simulink model "Dynamics"  (R2023a)
settings: Solver=FixedStepAuto  StartTime=0.0  StopTime=inf  FixedStep=0.001  EnableMultiTasking=on
libraries: sharedutil x32, sharedtransform x18, dspmtrx3 x12, matrix_library x6, simulink_extras x1, simulink x1
(part 4 of 6)

== system Dynamics/Subsystem2/Jacobian/J(q) gen./J_v_2(q) ==
  R_1^0 : Inport
  p_1^0 : Inport  Port=2
  p_2^0 : Inport  Port=3
  type1 : Inport  Port=4
  Constant : Constant  Value=zeros(3,1)
  J_v_1 : Subsystem
  v2M_1 : MATLAB Function  TreatAsAtomicUnit=on
  v2M_2 : MATLAB Function  TreatAsAtomicUnit=on
  v2M_3 : MATLAB Function  TreatAsAtomicUnit=on
  v2M_4 : MATLAB Function  TreatAsAtomicUnit=on
  v2M_5 : MATLAB Function  TreatAsAtomicUnit=on
  J_v_2(q) : Outport
  wires:
  R_1^0/1 -> J_v_1/1(R)
  J_v_1/1(J_v) -> v2M_1/1(v1)
  v2M_1/1(M) -> v2M_2/1(v1)
  v2M_2/1(M) -> v2M_3/1(v1)
  v2M_3/1(M) -> v2M_4/1(v1)
  v2M_4/1(M) -> v2M_5/1(v1)
  v2M_5/1(M) -> J_v_2(q)/1
  Constant/1 -> v2M_3/2(v2), v2M_4/2(v2), v2M_5/2(v2), v2M_1/2(v2), v2M_2/2(v2)
  p_1^0/1 -> J_v_1/2(p)
  type1/1 -> J_v_1/4(type)
  p_2^0/1 -> J_v_1/3(pn)

== system Dynamics/Subsystem2/Jacobian/J(q) gen./J_v_3(q) ==
  R_1^0 : Inport
  R_2^0 : Inport  Port=2
  p_1^0 : Inport  Port=3
  p_2^0 : Inport  Port=4
  p_3^0 : Inport  Port=5
  type1 : Inport  Port=6
  type2 : Inport  Port=7
  Constant : Constant  Value=zeros(3,1)
  J_v_1 : Subsystem
  J_v_2 : Subsystem
  v2M_1 : MATLAB Function  TreatAsAtomicUnit=on
  v2M_2 : MATLAB Function  TreatAsAtomicUnit=on
  v2M_3 : MATLAB Function  TreatAsAtomicUnit=on
  v2M_4 : MATLAB Function  TreatAsAtomicUnit=on
  v2M_5 : MATLAB Function  TreatAsAtomicUnit=on
  J_v_3(q) : Outport
  wires:
  R_1^0/1 -> J_v_1/1(R)
  J_v_1/1(J_v) -> v2M_1/1(v1)
  v2M_1/1(M) -> v2M_2/1(v1)
  v2M_2/1(M) -> v2M_3/1(v1)
  v2M_3/1(M) -> v2M_4/1(v1)
  v2M_4/1(M) -> v2M_5/1(v1)
  v2M_5/1(M) -> J_v_3(q)/1
  J_v_2/1(J_v) -> v2M_1/2(v2)
  Constant/1 -> v2M_5/2(v2), v2M_4/2(v2), v2M_2/2(v2), v2M_3/2(v2)
  R_2^0/1 -> J_v_2/1(R)
  p_1^0/1 -> J_v_1/2(p)
  p_2^0/1 -> J_v_2/2(p)
  type2/1 -> J_v_2/4(type)
  type1/1 -> J_v_1/4(type)
  p_3^0/1 -> J_v_1/3(pn), J_v_2/3(pn)

== system Dynamics/Subsystem2/Jacobian/J(q) gen./J_v_4(q) ==
  R_1^0 : Inport
  R_2^0 : Inport  Port=2
  R_3^0 : Inport  Port=3
  p_1^0 : Inport  Port=4
  p_2^0 : Inport  Port=5
  p_3^0 : Inport  Port=6
  p_4^0 : Inport  Port=7
  type1 : Inport  Port=8
  type2 : Inport  Port=9
  type3 : Inport  Port=10
  Constant : Constant  Value=zeros(3,1)
  J_v_1 : Subsystem
  J_v_2 : Subsystem
  J_v_3 : Subsystem
  v2M_1 : MATLAB Function  TreatAsAtomicUnit=on
  v2M_2 : MATLAB Function  TreatAsAtomicUnit=on
  v2M_3 : MATLAB Function  TreatAsAtomicUnit=on
  v2M_4 : MATLAB Function  TreatAsAtomicUnit=on
  v2M_5 : MATLAB Function  TreatAsAtomicUnit=on
  J_v_4(q) : Outport
  wires:
  R_1^0/1 -> J_v_1/1(R)
  J_v_1/1(J_v) -> v2M_1/1(v1)
  v2M_1/1(M) -> v2M_2/1(v1)
  v2M_2/1(M) -> v2M_3/1(v1)
  v2M_3/1(M) -> v2M_4/1(v1)
  v2M_4/1(M) -> v2M_5/1(v1)
  v2M_5/1(M) -> J_v_4(q)/1
  J_v_2/1(J_v) -> v2M_1/2(v2)
  J_v_3/1(J_v) -> v2M_2/2(v2)
  Constant/1 -> v2M_5/2(v2), v2M_3/2(v2), v2M_4/2(v2)
  R_2^0/1 -> J_v_2/1(R)
  R_3^0/1 -> J_v_3/1(R)
  p_1^0/1 -> J_v_1/2(p)
  p_2^0/1 -> J_v_2/2(p)
  p_3^0/1 -> J_v_3/2(p)
  type2/1 -> J_v_2/4(type)
  type1/1 -> J_v_1/4(type)
  type3/1 -> J_v_3/4(type)
  p_4^0/1 -> J_v_1/3(pn), J_v_2/3(pn), J_v_3/3(pn)

== system Dynamics/Subsystem2/Jacobian/J(q) gen./J_v_5(q) ==
  R_1^0 : Inport
  R_2^0 : Inport  Port=2
  R_3^0 : Inport  Port=3
  R_4^0 : Inport  Port=4
  p_1^0 : Inport  Port=5
  p_2^0 : Inport  Port=6
  p_3^0 : Inport  Port=7
  p_4^0 : Inport  Port=8
  p_5^0 : Inport  Port=9
  type1 : Inport  Port=10
  type2 : Inport  Port=11
  type3 : Inport  Port=12
  type4 : Inport  Port=13
  Constant : Constant  Value=zeros(3,1)
  J_v_1 : Subsystem
  J_v_2 : Subsystem
  J_v_3 : Subsystem
  J_v_4 : Subsystem
  v2M_1 : MATLAB Function  TreatAsAtomicUnit=on
  v2M_2 : MATLAB Function  TreatAsAtomicUnit=on
  v2M_3 : MATLAB Function  TreatAsAtomicUnit=on
  v2M_4 : MATLAB Function  TreatAsAtomicUnit=on
  v2M_5 : MATLAB Function  TreatAsAtomicUnit=on
  J_v_5(q) : Outport
  wires:
  R_1^0/1 -> J_v_1/1(R)
  J_v_1/1(J_v) -> v2M_1/1(v1)
  v2M_1/1(M) -> v2M_2/1(v1)
  v2M_2/1(M) -> v2M_3/1(v1)
  v2M_3/1(M) -> v2M_4/1(v1)
  v2M_4/1(M) -> v2M_5/1(v1)
  v2M_5/1(M) -> J_v_5(q)/1
  J_v_2/1(J_v) -> v2M_1/2(v2)
  J_v_3/1(J_v) -> v2M_2/2(v2)
  J_v_4/1(J_v) -> v2M_3/2(v2)
  Constant/1 -> v2M_4/2(v2), v2M_5/2(v2)
  R_2^0/1 -> J_v_2/1(R)
  R_3^0/1 -> J_v_3/1(R)
  R_4^0/1 -> J_v_4/1(R)
  p_1^0/1 -> J_v_1/2(p)
  p_2^0/1 -> J_v_2/2(p)
  p_3^0/1 -> J_v_3/2(p)
  p_4^0/1 -> J_v_4/2(p)
  type2/1 -> J_v_2/4(type)
  type1/1 -> J_v_1/4(type)
  type3/1 -> J_v_3/4(type)
  type4/1 -> J_v_4/4(type)
  p_5^0/1 -> J_v_1/3(pn), J_v_2/3(pn), J_v_3/3(pn), J_v_4/3(pn)

== system Dynamics/Subsystem2/Jacobian/J_v/J_v_1 ==
  R : Inport
  p : Inport  Port=2
  pn : Inport  Port=3
  type : Inport  Port=4
  Add : Sum
  If : If  IfExpression=u1 == 1
  Prismatic Action : Subsystem  TreatAsAtomicUnit=on
  Revolute Action : Subsystem  TreatAsAtomicUnit=on
  J_v : Outport
  wires:
  type/1 -> If/1
  If/1 -> Revolute Action/Action
  If/2 -> Prismatic Action/Action
  Revolute Action/1(J_v) -> Add/1
  Prismatic Action/1(J_v) -> Add/2
  Add/1 -> J_v/1
  R/1 -> Prismatic Action/1(R), Revolute Action/1(R)
  p/1 -> Revolute Action/2(p)
  pn/1 -> Revolute Action/3(pn)

== system Dynamics/Subsystem2/Jacobian/J_v/J_v_2 ==
  R : Inport
  p : Inport  Port=2
  pn : Inport  Port=3
  type : Inport  Port=4
  Add : Sum
  If : If  IfExpression=u1 == 1
  Prismatic Action : Subsystem  TreatAsAtomicUnit=on
  Revolute Action : Subsystem  TreatAsAtomicUnit=on
  J_v : Outport
  wires:
  type/1 -> If/1
  If/1 -> Revolute Action/Action
  If/2 -> Prismatic Action/Action
  Revolute Action/1(J_v) -> Add/1
  Prismatic Action/1(J_v) -> Add/2
  Add/1 -> J_v/1
  R/1 -> Prismatic Action/1(R), Revolute Action/1(R)
  p/1 -> Revolute Action/2(p)
  pn/1 -> Revolute Action/3(pn)

== system Dynamics/Subsystem2/Jacobian/J_v/J_v_3 ==
  R : Inport
  p : Inport  Port=2
  pn : Inport  Port=3
  type : Inport  Port=4
  Add : Sum
  If : If  IfExpression=u1 == 1
  Prismatic Action : Subsystem  TreatAsAtomicUnit=on
  Revolute Action : Subsystem  TreatAsAtomicUnit=on
  J_v : Outport
  wires:
  type/1 -> If/1
  If/1 -> Revolute Action/Action
  If/2 -> Prismatic Action/Action
  Revolute Action/1(J_v) -> Add/1
  Prismatic Action/1(J_v) -> Add/2
  Add/1 -> J_v/1
  R/1 -> Prismatic Action/1(R), Revolute Action/1(R)
  p/1 -> Revolute Action/2(p)
  pn/1 -> Revolute Action/3(pn)

== system Dynamics/Subsystem2/Jacobian/J_v/J_v_4 ==
  R : Inport
  p : Inport  Port=2
  pn : Inport  Port=3
  type : Inport  Port=4
  Add : Sum
  If : If  IfExpression=u1 == 1
  Prismatic Action : Subsystem  TreatAsAtomicUnit=on
  Revolute Action : Subsystem  TreatAsAtomicUnit=on
  J_v : Outport
  wires:
  type/1 -> If/1
  If/1 -> Revolute Action/Action
  If/2 -> Prismatic Action/Action
  Revolute Action/1(J_v) -> Add/1
  Prismatic Action/1(J_v) -> Add/2
  Add/1 -> J_v/1
  R/1 -> Prismatic Action/1(R), Revolute Action/1(R)
  p/1 -> Revolute Action/2(p)
  pn/1 -> Revolute Action/3(pn)

== system Dynamics/Subsystem2/Jacobian/J_v/J_v_5 ==
  R : Inport
  p : Inport  Port=2
  pn : Inport  Port=3
  type : Inport  Port=4
  Add : Sum
  If : If  IfExpression=u1 == 1
  Prismatic Action : Subsystem  TreatAsAtomicUnit=on
  Revolute Action : Subsystem  TreatAsAtomicUnit=on
  J_v : Outport
  wires:
  type/1 -> If/1
  If/1 -> Revolute Action/Action
  If/2 -> Prismatic Action/Action
  Revolute Action/1(J_v) -> Add/1
  Prismatic Action/1(J_v) -> Add/2
  Add/1 -> J_v/1
  R/1 -> Prismatic Action/1(R), Revolute Action/1(R)
  p/1 -> Revolute Action/2(p)
  pn/1 -> Revolute Action/3(pn)

== system Dynamics/Subsystem2/Jacobian/J_v/J_v_6 ==
  R : Inport
  p : Inport  Port=2
  pn : Inport  Port=3
  type : Inport  Port=4
  Add : Sum
  If : If  IfExpression=u1 == 1
  Prismatic Action : Subsystem  TreatAsAtomicUnit=on
  Revolute Action : Subsystem  TreatAsAtomicUnit=on
  J_v : Outport
  wires:
  type/1 -> If/1
  If/1 -> Revolute Action/Action
  If/2 -> Prismatic Action/Action
  Revolute Action/1(J_v) -> Add/1
  Prismatic Action/1(J_v) -> Add/2
  Add/1 -> J_v/1
  R/1 -> Prismatic Action/1(R), Revolute Action/1(R)
  p/1 -> Revolute Action/2(p)
  pn/1 -> Revolute Action/3(pn)

== system Dynamics/DYNAMIC/Jacobian/J(q) gen./J_v_2(q)/J_v_1 ==
  R : Inport
  p : Inport  Port=2
  pn : Inport  Port=3
  type : Inport  Port=4
  Add : Sum
  If : If  IfExpression=u1 == 1
  Prismatic Action : Subsystem  TreatAsAtomicUnit=on
  Revolute Action : Subsystem  TreatAsAtomicUnit=on
  J_v : Outport
  wires:
  type/1 -> If/1
  If/1 -> Revolute Action/Action
  If/2 -> Prismatic Action/Action
  Revolute Action/1(J_v) -> Add/1
  Prismatic Action/1(J_v) -> Add/2
  Add/1 -> J_v/1
  R/1 -> Prismatic Action/1(R), Revolute Action/1(R)
  p/1 -> Revolute Action/2(p)
  pn/1 -> Revolute Action/3(pn)

== system Dynamics/DYNAMIC/Jacobian/J(q) gen./J_v_3(q)/J_v_1 ==
  R : Inport
  p : Inport  Port=2
  pn : Inport  Port=3
  type : Inport  Port=4
  Add : Sum
  If : If  IfExpression=u1 == 1
  Prismatic Action : Subsystem  TreatAsAtomicUnit=on
  Revolute Action : Subsystem  TreatAsAtomicUnit=on
  J_v : Outport
  wires:
  type/1 -> If/1
  If/1 -> Revolute Action/Action
  If/2 -> Prismatic Action/Action
  Revolute Action/1(J_v) -> Add/1
  Prismatic Action/1(J_v) -> Add/2
  Add/1 -> J_v/1
  R/1 -> Prismatic Action/1(R), Revolute Action/1(R)
  p/1 -> Revolute Action/2(p)
  pn/1 -> Revolute Action/3(pn)

== system Dynamics/DYNAMIC/Jacobian/J(q) gen./J_v_3(q)/J_v_2 ==
  R : Inport
  p : Inport  Port=2
  pn : Inport  Port=3
  type : Inport  Port=4
  Add : Sum
  If : If  IfExpression=u1 == 1
  Prismatic Action : Subsystem  TreatAsAtomicUnit=on
  Revolute Action : Subsystem  TreatAsAtomicUnit=on
  J_v : Outport
  wires:
  type/1 -> If/1
  If/1 -> Revolute Action/Action
  If/2 -> Prismatic Action/Action
  Revolute Action/1(J_v) -> Add/1
  Prismatic Action/1(J_v) -> Add/2
  Add/1 -> J_v/1
  R/1 -> Prismatic Action/1(R), Revolute Action/1(R)
  p/1 -> Revolute Action/2(p)
  pn/1 -> Revolute Action/3(pn)

== system Dynamics/DYNAMIC/Jacobian/J(q) gen./J_v_4(q)/J_v_1 ==
  R : Inport
  p : Inport  Port=2
  pn : Inport  Port=3
  type : Inport  Port=4
  Add : Sum
  If : If  IfExpression=u1 == 1
  Prismatic Action : Subsystem  TreatAsAtomicUnit=on
  Revolute Action : Subsystem  TreatAsAtomicUnit=on
  J_v : Outport
  wires:
  type/1 -> If/1
  If/1 -> Revolute Action/Action
  If/2 -> Prismatic Action/Action
  Revolute Action/1(J_v) -> Add/1
  Prismatic Action/1(J_v) -> Add/2
  Add/1 -> J_v/1
  R/1 -> Prismatic Action/1(R), Revolute Action/1(R)
  p/1 -> Revolute Action/2(p)
  pn/1 -> Revolute Action/3(pn)

== system Dynamics/DYNAMIC/Jacobian/J(q) gen./J_v_4(q)/J_v_2 ==
  R : Inport
  p : Inport  Port=2
  pn : Inport  Port=3
  type : Inport  Port=4
  Add : Sum
  If : If  IfExpression=u1 == 1
  Prismatic Action : Subsystem  TreatAsAtomicUnit=on
  Revolute Action : Subsystem  TreatAsAtomicUnit=on
  J_v : Outport
  wires:
  type/1 -> If/1
  If/1 -> Revolute Action/Action
  If/2 -> Prismatic Action/Action
  Revolute Action/1(J_v) -> Add/1
  Prismatic Action/1(J_v) -> Add/2
  Add/1 -> J_v/1
  R/1 -> Prismatic Action/1(R), Revolute Action/1(R)
  p/1 -> Revolute Action/2(p)
  pn/1 -> Revolute Action/3(pn)

== system Dynamics/DYNAMIC/Jacobian/J(q) gen./J_v_4(q)/J_v_3 ==
  R : Inport
  p : Inport  Port=2
  pn : Inport  Port=3
  type : Inport  Port=4
  Add : Sum
  If : If  IfExpression=u1 == 1
  Prismatic Action : Subsystem  TreatAsAtomicUnit=on
  Revolute Action : Subsystem  TreatAsAtomicUnit=on
  J_v : Outport
  wires:
  type/1 -> If/1
  If/1 -> Revolute Action/Action
  If/2 -> Prismatic Action/Action
  Revolute Action/1(J_v) -> Add/1
  Prismatic Action/1(J_v) -> Add/2
  Add/1 -> J_v/1
  R/1 -> Prismatic Action/1(R), Revolute Action/1(R)
  p/1 -> Revolute Action/2(p)
  pn/1 -> Revolute Action/3(pn)

== system Dynamics/DYNAMIC/Jacobian/J(q) gen./J_v_5(q)/J_v_1 ==
  R : Inport
  p : Inport  Port=2
  pn : Inport  Port=3
  type : Inport  Port=4
  Add : Sum
  If : If  IfExpression=u1 == 1
  Prismatic Action : Subsystem  TreatAsAtomicUnit=on
  Revolute Action : Subsystem  TreatAsAtomicUnit=on
  J_v : Outport
  wires:
  type/1 -> If/1
  If/1 -> Revolute Action/Action
  If/2 -> Prismatic Action/Action
  Revolute Action/1(J_v) -> Add/1
  Prismatic Action/1(J_v) -> Add/2
  Add/1 -> J_v/1
  R/1 -> Prismatic Action/1(R), Revolute Action/1(R)
  p/1 -> Revolute Action/2(p)
  pn/1 -> Revolute Action/3(pn)

== system Dynamics/DYNAMIC/Jacobian/J(q) gen./J_v_5(q)/J_v_2 ==
  R : Inport
  p : Inport  Port=2
  pn : Inport  Port=3
  type : Inport  Port=4
  Add : Sum
  If : If  IfExpression=u1 == 1
  Prismatic Action : Subsystem  TreatAsAtomicUnit=on
  Revolute Action : Subsystem  TreatAsAtomicUnit=on
  J_v : Outport
  wires:
  type/1 -> If/1
  If/1 -> Revolute Action/Action
  If/2 -> Prismatic Action/Action
  Revolute Action/1(J_v) -> Add/1
  Prismatic Action/1(J_v) -> Add/2
  Add/1 -> J_v/1
  R/1 -> Prismatic Action/1(R), Revolute Action/1(R)
  p/1 -> Revolute Action/2(p)
  pn/1 -> Revolute Action/3(pn)

== system Dynamics/DYNAMIC/Jacobian/J(q) gen./J_v_5(q)/J_v_3 ==
  R : Inport
  p : Inport  Port=2
  pn : Inport  Port=3
  type : Inport  Port=4
  Add : Sum
  If : If  IfExpression=u1 == 1
  Prismatic Action : Subsystem  TreatAsAtomicUnit=on
  Revolute Action : Subsystem  TreatAsAtomicUnit=on
  J_v : Outport
  wires:
  type/1 -> If/1
  If/1 -> Revolute Action/Action
  If/2 -> Prismatic Action/Action
  Revolute Action/1(J_v) -> Add/1
  Prismatic Action/1(J_v) -> Add/2
  Add/1 -> J_v/1
  R/1 -> Prismatic Action/1(R), Revolute Action/1(R)
  p/1 -> Revolute Action/2(p)
  pn/1 -> Revolute Action/3(pn)

== system Dynamics/DYNAMIC/Jacobian/J(q) gen./J_v_5(q)/J_v_4 ==
  R : Inport
  p : Inport  Port=2
  pn : Inport  Port=3
  type : Inport  Port=4
  Add : Sum
  If : If  IfExpression=u1 == 1
  Prismatic Action : Subsystem  TreatAsAtomicUnit=on
  Revolute Action : Subsystem  TreatAsAtomicUnit=on
  J_v : Outport
  wires:
  type/1 -> If/1
  If/1 -> Revolute Action/Action
  If/2 -> Prismatic Action/Action
  Revolute Action/1(J_v) -> Add/1
  Prismatic Action/1(J_v) -> Add/2
  Add/1 -> J_v/1
  R/1 -> Prismatic Action/1(R), Revolute Action/1(R)
  p/1 -> Revolute Action/2(p)
  pn/1 -> Revolute Action/3(pn)

== system Dynamics/DYNAMIC/Jacobian/J_v/J_v_1/Prismatic Action ==
  R : Inport
  Action Port : ActionPort  ActionPortLabel=else
  Constant : Constant  Value=[0;0;1]
  Product : Product  Multiplication=Matrix(*)
  J_v : Outport
  wires:
  Product/1 -> J_v/1
  R/1 -> Product/1
  Constant/1 -> Product/2

== system Dynamics/DYNAMIC/Jacobian/J_v/J_v_1/Revolute Action ==
  R : Inport
  p : Inport  Port=2
  pn : Inport  Port=3
  Action Port : ActionPort  ActionPortLabel=if(u1 == 1)
  3x3 Cross Product : sharedutil/3x3 Cross Product  aMode=aMode
  Add : Sum  Inputs=-+
  Constant : Constant  Value=[0;0;1]
  Product : Product  Multiplication=Matrix(*)
  J_v : Outport
  wires:
  3x3 Cross Product/1 -> J_v/1
  p/1 -> Add/1
  pn/1 -> Add/2
  Add/1 -> 3x3 Cross Product/2
  R/1 -> Product/1
  Constant/1 -> Product/2
  Product/1 -> 3x3 Cross Product/1

== system Dynamics/DYNAMIC/Jacobian/J_v/J_v_2/Prismatic Action ==
  R : Inport
  Action Port : ActionPort  ActionPortLabel=else
  Constant : Constant  Value=[0;0;1]
  Product : Product  Multiplication=Matrix(*)
  J_v : Outport
  wires:
  Product/1 -> J_v/1
  R/1 -> Product/1
  Constant/1 -> Product/2

== system Dynamics/DYNAMIC/Jacobian/J_v/J_v_2/Revolute Action ==
  R : Inport
  p : Inport  Port=2
  pn : Inport  Port=3
  Action Port : ActionPort  ActionPortLabel=if(u1 == 1)
  3x3 Cross Product : sharedutil/3x3 Cross Product  aMode=aMode
  Add : Sum  Inputs=-+
  Constant : Constant  Value=[0;0;1]
  Product : Product  Multiplication=Matrix(*)
  J_v : Outport
  wires:
  3x3 Cross Product/1 -> J_v/1
  p/1 -> Add/1
  pn/1 -> Add/2
  Add/1 -> 3x3 Cross Product/2
  R/1 -> Product/1
  Constant/1 -> Product/2
  Product/1 -> 3x3 Cross Product/1

== system Dynamics/DYNAMIC/Jacobian/J_v/J_v_3/Prismatic Action ==
  R : Inport
  Action Port : ActionPort  ActionPortLabel=else
  Constant : Constant  Value=[0;0;1]
  Product : Product  Multiplication=Matrix(*)
  J_v : Outport
  wires:
  Product/1 -> J_v/1
  R/1 -> Product/1
  Constant/1 -> Product/2

== system Dynamics/DYNAMIC/Jacobian/J_v/J_v_3/Revolute Action ==
  R : Inport
  p : Inport  Port=2
  pn : Inport  Port=3
  Action Port : ActionPort  ActionPortLabel=if(u1 == 1)
  3x3 Cross Product : sharedutil/3x3 Cross Product  aMode=aMode
  Add : Sum  Inputs=-+
  Constant : Constant  Value=[0;0;1]
  Product : Product  Multiplication=Matrix(*)
  J_v : Outport
  wires:
  3x3 Cross Product/1 -> J_v/1
  p/1 -> Add/1
  pn/1 -> Add/2
  Add/1 -> 3x3 Cross Product/2
  R/1 -> Product/1
  Constant/1 -> Product/2
  Product/1 -> 3x3 Cross Product/1

== system Dynamics/DYNAMIC/Jacobian/J_v/J_v_4/Prismatic Action ==
  R : Inport
  Action Port : ActionPort  ActionPortLabel=else
  Constant : Constant  Value=[0;0;1]
  Product : Product  Multiplication=Matrix(*)
  J_v : Outport
  wires:
  Product/1 -> J_v/1
  R/1 -> Product/1
  Constant/1 -> Product/2

== system Dynamics/DYNAMIC/Jacobian/J_v/J_v_4/Revolute Action ==
  R : Inport
  p : Inport  Port=2
  pn : Inport  Port=3
  Action Port : ActionPort  ActionPortLabel=if(u1 == 1)
  3x3 Cross Product : sharedutil/3x3 Cross Product  aMode=aMode
  Add : Sum  Inputs=-+
  Constant : Constant  Value=[0;0;1]
  Product : Product  Multiplication=Matrix(*)
  J_v : Outport
  wires:
  3x3 Cross Product/1 -> J_v/1
  p/1 -> Add/1
  pn/1 -> Add/2
  Add/1 -> 3x3 Cross Product/2
  R/1 -> Product/1
  Constant/1 -> Product/2
  Product/1 -> 3x3 Cross Product/1

== system Dynamics/DYNAMIC/Jacobian/J_v/J_v_5/Prismatic Action ==
  R : Inport
  Action Port : ActionPort  ActionPortLabel=else
  Constant : Constant  Value=[0;0;1]
  Product : Product  Multiplication=Matrix(*)
  J_v : Outport
  wires:
  Product/1 -> J_v/1
  R/1 -> Product/1
  Constant/1 -> Product/2

== system Dynamics/DYNAMIC/Jacobian/J_v/J_v_5/Revolute Action ==
  R : Inport
  p : Inport  Port=2
  pn : Inport  Port=3
  Action Port : ActionPort  ActionPortLabel=if(u1 == 1)
  3x3 Cross Product : sharedutil/3x3 Cross Product  aMode=aMode
  Add : Sum  Inputs=-+
  Constant : Constant  Value=[0;0;1]
  Product : Product  Multiplication=Matrix(*)
  J_v : Outport
  wires:
  3x3 Cross Product/1 -> J_v/1
  p/1 -> Add/1
  pn/1 -> Add/2
  Add/1 -> 3x3 Cross Product/2
  R/1 -> Product/1
  Constant/1 -> Product/2
  Product/1 -> 3x3 Cross Product/1

== system Dynamics/DYNAMIC/Jacobian/J_v/J_v_6/Prismatic Action ==
  R : Inport
  Action Port : ActionPort  ActionPortLabel=else
  Constant : Constant  Value=[0;0;1]
  Product : Product  Multiplication=Matrix(*)
  J_v : Outport
  wires:
  Product/1 -> J_v/1
  R/1 -> Product/1
  Constant/1 -> Product/2

== system Dynamics/DYNAMIC/Jacobian/J_v/J_v_6/Revolute Action ==
  R : Inport
  p : Inport  Port=2
  pn : Inport  Port=3
  Action Port : ActionPort  ActionPortLabel=if(u1 == 1)
  3x3 Cross Product : sharedutil/3x3 Cross Product  aMode=aMode
  Add : Sum  Inputs=-+
  Constant : Constant  Value=[0;0;1]
  Product : Product  Multiplication=Matrix(*)
  J_v : Outport
  wires:
  3x3 Cross Product/1 -> J_v/1
  p/1 -> Add/1
  pn/1 -> Add/2
  Add/1 -> 3x3 Cross Product/2
  R/1 -> Product/1
  Constant/1 -> Product/2
  Product/1 -> 3x3 Cross Product/1

== system Dynamics/Subsystem/Jacobian/J(q) gen./J_v_2(q)/J_v_1 ==
  R : Inport
  p : Inport  Port=2
  pn : Inport  Port=3
  type : Inport  Port=4
  Add : Sum
  If : If  IfExpression=u1 == 1
  Prismatic Action : Subsystem  TreatAsAtomicUnit=on
  Revolute Action : Subsystem  TreatAsAtomicUnit=on
  J_v : Outport
  wires:
  type/1 -> If/1
  If/1 -> Revolute Action/Action
  If/2 -> Prismatic Action/Action
  Revolute Action/1(J_v) -> Add/1
  Prismatic Action/1(J_v) -> Add/2
  Add/1 -> J_v/1
  R/1 -> Prismatic Action/1(R), Revolute Action/1(R)
  p/1 -> Revolute Action/2(p)
  pn/1 -> Revolute Action/3(pn)

== system Dynamics/Subsystem/Jacobian/J(q) gen./J_v_3(q)/J_v_1 ==
  R : Inport
  p : Inport  Port=2
  pn : Inport  Port=3
  type : Inport  Port=4
  Add : Sum
  If : If  IfExpression=u1 == 1
  Prismatic Action : Subsystem  TreatAsAtomicUnit=on
  Revolute Action : Subsystem  TreatAsAtomicUnit=on
  J_v : Outport
  wires:
  type/1 -> If/1
  If/1 -> Revolute Action/Action
  If/2 -> Prismatic Action/Action
  Revolute Action/1(J_v) -> Add/1
  Prismatic Action/1(J_v) -> Add/2
  Add/1 -> J_v/1
  R/1 -> Prismatic Action/1(R), Revolute Action/1(R)
  p/1 -> Revolute Action/2(p)
  pn/1 -> Revolute Action/3(pn)

== system Dynamics/Subsystem/Jacobian/J(q) gen./J_v_3(q)/J_v_2 ==
  R : Inport
  p : Inport  Port=2
  pn : Inport  Port=3
  type : Inport  Port=4
  Add : Sum
  If : If  IfExpression=u1 == 1
  Prismatic Action : Subsystem  TreatAsAtomicUnit=on
  Revolute Action : Subsystem  TreatAsAtomicUnit=on
  J_v : Outport
  wires:
  type/1 -> If/1
  If/1 -> Revolute Action/Action
  If/2 -> Prismatic Action/Action
  Revolute Action/1(J_v) -> Add/1
  Prismatic Action/1(J_v) -> Add/2
  Add/1 -> J_v/1
  R/1 -> Prismatic Action/1(R), Revolute Action/1(R)
  p/1 -> Revolute Action/2(p)
  pn/1 -> Revolute Action/3(pn)

== system Dynamics/Subsystem/Jacobian/J(q) gen./J_v_4(q)/J_v_1 ==
  R : Inport
  p : Inport  Port=2
  pn : Inport  Port=3
  type : Inport  Port=4
  Add : Sum
  If : If  IfExpression=u1 == 1
  Prismatic Action : Subsystem  TreatAsAtomicUnit=on
  Revolute Action : Subsystem  TreatAsAtomicUnit=on
  J_v : Outport
  wires:
  type/1 -> If/1
  If/1 -> Revolute Action/Action
  If/2 -> Prismatic Action/Action
  Revolute Action/1(J_v) -> Add/1
  Prismatic Action/1(J_v) -> Add/2
  Add/1 -> J_v/1
  R/1 -> Prismatic Action/1(R), Revolute Action/1(R)
  p/1 -> Revolute Action/2(p)
  pn/1 -> Revolute Action/3(pn)

== system Dynamics/Subsystem/Jacobian/J(q) gen./J_v_4(q)/J_v_2 ==
  R : Inport
  p : Inport  Port=2
  pn : Inport  Port=3
  type : Inport  Port=4
  Add : Sum
  If : If  IfExpression=u1 == 1
  Prismatic Action : Subsystem  TreatAsAtomicUnit=on
  Revolute Action : Subsystem  TreatAsAtomicUnit=on
  J_v : Outport
  wires:
  type/1 -> If/1
  If/1 -> Revolute Action/Action
  If/2 -> Prismatic Action/Action
  Revolute Action/1(J_v) -> Add/1
  Prismatic Action/1(J_v) -> Add/2
  Add/1 -> J_v/1
  R/1 -> Prismatic Action/1(R), Revolute Action/1(R)
  p/1 -> Revolute Action/2(p)
  pn/1 -> Revolute Action/3(pn)

== system Dynamics/Subsystem/Jacobian/J(q) gen./J_v_4(q)/J_v_3 ==
  R : Inport
  p : Inport  Port=2
  pn : Inport  Port=3
  type : Inport  Port=4
  Add : Sum
  If : If  IfExpression=u1 == 1
  Prismatic Action : Subsystem  TreatAsAtomicUnit=on
  Revolute Action : Subsystem  TreatAsAtomicUnit=on
  J_v : Outport
  wires:
  type/1 -> If/1
  If/1 -> Revolute Action/Action
  If/2 -> Prismatic Action/Action
  Revolute Action/1(J_v) -> Add/1
  Prismatic Action/1(J_v) -> Add/2
  Add/1 -> J_v/1
  R/1 -> Prismatic Action/1(R), Revolute Action/1(R)
  p/1 -> Revolute Action/2(p)
  pn/1 -> Revolute Action/3(pn)

== system Dynamics/Subsystem/Jacobian/J(q) gen./J_v_5(q)/J_v_1 ==
  R : Inport
  p : Inport  Port=2
  pn : Inport  Port=3
  type : Inport  Port=4
  Add : Sum
  If : If  IfExpression=u1 == 1
  Prismatic Action : Subsystem  TreatAsAtomicUnit=on
  Revolute Action : Subsystem  TreatAsAtomicUnit=on
  J_v : Outport
  wires:
  type/1 -> If/1
  If/1 -> Revolute Action/Action
  If/2 -> Prismatic Action/Action
  Revolute Action/1(J_v) -> Add/1
  Prismatic Action/1(J_v) -> Add/2
  Add/1 -> J_v/1
  R/1 -> Prismatic Action/1(R), Revolute Action/1(R)
  p/1 -> Revolute Action/2(p)
  pn/1 -> Revolute Action/3(pn)

== system Dynamics/Subsystem/Jacobian/J(q) gen./J_v_5(q)/J_v_2 ==
  R : Inport
  p : Inport  Port=2
  pn : Inport  Port=3
  type : Inport  Port=4
  Add : Sum
  If : If  IfExpression=u1 == 1
  Prismatic Action : Subsystem  TreatAsAtomicUnit=on
  Revolute Action : Subsystem  TreatAsAtomicUnit=on
  J_v : Outport
  wires:
  type/1 -> If/1
  If/1 -> Revolute Action/Action
  If/2 -> Prismatic Action/Action
  Revolute Action/1(J_v) -> Add/1
  Prismatic Action/1(J_v) -> Add/2
  Add/1 -> J_v/1
  R/1 -> Prismatic Action/1(R), Revolute Action/1(R)
  p/1 -> Revolute Action/2(p)
  pn/1 -> Revolute Action/3(pn)

== system Dynamics/Subsystem/Jacobian/J(q) gen./J_v_5(q)/J_v_3 ==
  R : Inport
  p : Inport  Port=2
  pn : Inport  Port=3
  type : Inport  Port=4
  Add : Sum
  If : If  IfExpression=u1 == 1
  Prismatic Action : Subsystem  TreatAsAtomicUnit=on
  Revolute Action : Subsystem  TreatAsAtomicUnit=on
  J_v : Outport
  wires:
  type/1 -> If/1
  If/1 -> Revolute Action/Action
  If/2 -> Prismatic Action/Action
  Revolute Action/1(J_v) -> Add/1
  Prismatic Action/1(J_v) -> Add/2
  Add/1 -> J_v/1
  R/1 -> Prismatic Action/1(R), Revolute Action/1(R)
  p/1 -> Revolute Action/2(p)
  pn/1 -> Revolute Action/3(pn)

== system Dynamics/Subsystem/Jacobian/J(q) gen./J_v_5(q)/J_v_4 ==
  R : Inport
  p : Inport  Port=2
  pn : Inport  Port=3
  type : Inport  Port=4
  Add : Sum
  If : If  IfExpression=u1 == 1
  Prismatic Action : Subsystem  TreatAsAtomicUnit=on
  Revolute Action : Subsystem  TreatAsAtomicUnit=on
  J_v : Outport
  wires:
  type/1 -> If/1
  If/1 -> Revolute Action/Action
  If/2 -> Prismatic Action/Action
  Revolute Action/1(J_v) -> Add/1
  Prismatic Action/1(J_v) -> Add/2
  Add/1 -> J_v/1
  R/1 -> Prismatic Action/1(R), Revolute Action/1(R)
  p/1 -> Revolute Action/2(p)
  pn/1 -> Revolute Action/3(pn)

== system Dynamics/Subsystem/Jacobian/J_v/J_v_1/Prismatic Action ==
  R : Inport
  Action Port : ActionPort  ActionPortLabel=else
  Constant : Constant  Value=[0;0;1]
  Product : Product  Multiplication=Matrix(*)
  J_v : Outport
  wires:
  Product/1 -> J_v/1
  R/1 -> Product/1
  Constant/1 -> Product/2

== system Dynamics/Subsystem/Jacobian/J_v/J_v_1/Revolute Action ==
  R : Inport
  p : Inport  Port=2
  pn : Inport  Port=3
  Action Port : ActionPort  ActionPortLabel=if(u1 == 1)
  3x3 Cross Product : sharedutil/3x3 Cross Product  aMode=aMode
  Add : Sum  Inputs=-+
  Constant : Constant  Value=[0;0;1]
  Product : Product  Multiplication=Matrix(*)
  J_v : Outport
  wires:
  3x3 Cross Product/1 -> J_v/1
  p/1 -> Add/1
  pn/1 -> Add/2
  Add/1 -> 3x3 Cross Product/2
  R/1 -> Product/1
  Constant/1 -> Product/2
  Product/1 -> 3x3 Cross Product/1

== system Dynamics/Subsystem/Jacobian/J_v/J_v_2/Prismatic Action ==
  R : Inport
  Action Port : ActionPort  ActionPortLabel=else
  Constant : Constant  Value=[0;0;1]
  Product : Product  Multiplication=Matrix(*)
  J_v : Outport
  wires:
  Product/1 -> J_v/1
  R/1 -> Product/1
  Constant/1 -> Product/2

== system Dynamics/Subsystem/Jacobian/J_v/J_v_2/Revolute Action ==
  R : Inport
  p : Inport  Port=2
  pn : Inport  Port=3
  Action Port : ActionPort  ActionPortLabel=if(u1 == 1)
  3x3 Cross Product : sharedutil/3x3 Cross Product  aMode=aMode
  Add : Sum  Inputs=-+
  Constant : Constant  Value=[0;0;1]
  Product : Product  Multiplication=Matrix(*)
  J_v : Outport
  wires:
  3x3 Cross Product/1 -> J_v/1
  p/1 -> Add/1
  pn/1 -> Add/2
  Add/1 -> 3x3 Cross Product/2
  R/1 -> Product/1
  Constant/1 -> Product/2
  Product/1 -> 3x3 Cross Product/1

== system Dynamics/Subsystem/Jacobian/J_v/J_v_3/Prismatic Action ==
  R : Inport
  Action Port : ActionPort  ActionPortLabel=else
  Constant : Constant  Value=[0;0;1]
  Product : Product  Multiplication=Matrix(*)
  J_v : Outport
  wires:
  Product/1 -> J_v/1
  R/1 -> Product/1
  Constant/1 -> Product/2

== system Dynamics/Subsystem/Jacobian/J_v/J_v_3/Revolute Action ==
  R : Inport
  p : Inport  Port=2
  pn : Inport  Port=3
  Action Port : ActionPort  ActionPortLabel=if(u1 == 1)
  3x3 Cross Product : sharedutil/3x3 Cross Product  aMode=aMode
  Add : Sum  Inputs=-+
  Constant : Constant  Value=[0;0;1]
  Product : Product  Multiplication=Matrix(*)
  J_v : Outport
  wires:
  3x3 Cross Product/1 -> J_v/1
  p/1 -> Add/1
  pn/1 -> Add/2
  Add/1 -> 3x3 Cross Product/2
  R/1 -> Product/1
  Constant/1 -> Product/2
  Product/1 -> 3x3 Cross Product/1

== system Dynamics/Subsystem/Jacobian/J_v/J_v_4/Prismatic Action ==
  R : Inport
  Action Port : ActionPort  ActionPortLabel=else
  Constant : Constant  Value=[0;0;1]
  Product : Product  Multiplication=Matrix(*)
  J_v : Outport
  wires:
  Product/1 -> J_v/1
  R/1 -> Product/1
  Constant/1 -> Product/2

== system Dynamics/Subsystem/Jacobian/J_v/J_v_4/Revolute Action ==
  R : Inport
  p : Inport  Port=2
  pn : Inport  Port=3
  Action Port : ActionPort  ActionPortLabel=if(u1 == 1)
  3x3 Cross Product : sharedutil/3x3 Cross Product  aMode=aMode
  Add : Sum  Inputs=-+
  Constant : Constant  Value=[0;0;1]
  Product : Product  Multiplication=Matrix(*)
  J_v : Outport
  wires:
  3x3 Cross Product/1 -> J_v/1
  p/1 -> Add/1
  pn/1 -> Add/2
  Add/1 -> 3x3 Cross Product/2
  R/1 -> Product/1
  Constant/1 -> Product/2
  Product/1 -> 3x3 Cross Product/1

== system Dynamics/Subsystem/Jacobian/J_v/J_v_5/Prismatic Action ==
  R : Inport
  Action Port : ActionPort  ActionPortLabel=else
  Constant : Constant  Value=[0;0;1]
  Product : Product  Multiplication=Matrix(*)
  J_v : Outport
  wires:
  Product/1 -> J_v/1
  R/1 -> Product/1
  Constant/1 -> Product/2

== system Dynamics/Subsystem/Jacobian/J_v/J_v_5/Revolute Action ==
  R : Inport
  p : Inport  Port=2
  pn : Inport  Port=3
  Action Port : ActionPort  ActionPortLabel=if(u1 == 1)
  3x3 Cross Product : sharedutil/3x3 Cross Product  aMode=aMode
  Add : Sum  Inputs=-+
  Constant : Constant  Value=[0;0;1]
  Product : Product  Multiplication=Matrix(*)
  J_v : Outport
  wires:
  3x3 Cross Product/1 -> J_v/1
  p/1 -> Add/1
  pn/1 -> Add/2
  Add/1 -> 3x3 Cross Product/2
  R/1 -> Product/1
  Constant/1 -> Product/2
  Product/1 -> 3x3 Cross Product/1

== system Dynamics/Subsystem/Jacobian/J_v/J_v_6/Prismatic Action ==
  R : Inport
  Action Port : ActionPort  ActionPortLabel=else
  Constant : Constant  Value=[0;0;1]
  Product : Product  Multiplication=Matrix(*)
  J_v : Outport
  wires:
  Product/1 -> J_v/1
  R/1 -> Product/1
  Constant/1 -> Product/2

== system Dynamics/Subsystem/Jacobian/J_v/J_v_6/Revolute Action ==
  R : Inport
  p : Inport  Port=2
  pn : Inport  Port=3
  Action Port : ActionPort  ActionPortLabel=if(u1 == 1)
  3x3 Cross Product : sharedutil/3x3 Cross Product  aMode=aMode
  Add : Sum  Inputs=-+
  Constant : Constant  Value=[0;0;1]
  Product : Product  Multiplication=Matrix(*)
  J_v : Outport
  wires:
  3x3 Cross Product/1 -> J_v/1
  p/1 -> Add/1
  pn/1 -> Add/2
  Add/1 -> 3x3 Cross Product/2
  R/1 -> Product/1
  Constant/1 -> Product/2
  Product/1 -> 3x3 Cross Product/1

== system Dynamics/Subsystem2/Jacobian/J(q) gen./J_v_2(q)/J_v_1 ==
  R : Inport
  p : Inport  Port=2
  pn : Inport  Port=3
  type : Inport  Port=4
  Add : Sum
  If : If  IfExpression=u1 == 1
  Prismatic Action : Subsystem  TreatAsAtomicUnit=on
  Revolute Action : Subsystem  TreatAsAtomicUnit=on
  J_v : Outport
  wires:
  type/1 -> If/1
  If/1 -> Revolute Action/Action
  If/2 -> Prismatic Action/Action
  Revolute Action/1(J_v) -> Add/1
  Prismatic Action/1(J_v) -> Add/2
  Add/1 -> J_v/1
  R/1 -> Prismatic Action/1(R), Revolute Action/1(R)
  p/1 -> Revolute Action/2(p)
  pn/1 -> Revolute Action/3(pn)

== system Dynamics/Subsystem2/Jacobian/J(q) gen./J_v_3(q)/J_v_1 ==
  R : Inport
  p : Inport  Port=2
  pn : Inport  Port=3
  type : Inport  Port=4
  Add : Sum
  If : If  IfExpression=u1 == 1
  Prismatic Action : Subsystem  TreatAsAtomicUnit=on
  Revolute Action : Subsystem  TreatAsAtomicUnit=on
  J_v : Outport
  wires:
  type/1 -> If/1
  If/1 -> Revolute Action/Action
  If/2 -> Prismatic Action/Action
  Revolute Action/1(J_v) -> Add/1
  Prismatic Action/1(J_v) -> Add/2
  Add/1 -> J_v/1
  R/1 -> Prismatic Action/1(R), Revolute Action/1(R)
  p/1 -> Revolute Action/2(p)
  pn/1 -> Revolute Action/3(pn)

== system Dynamics/Subsystem2/Jacobian/J(q) gen./J_v_3(q)/J_v_2 ==
  R : Inport
  p : Inport  Port=2
  pn : Inport  Port=3
  type : Inport  Port=4
  Add : Sum
  If : If  IfExpression=u1 == 1
  Prismatic Action : Subsystem  TreatAsAtomicUnit=on
  Revolute Action : Subsystem  TreatAsAtomicUnit=on
  J_v : Outport
  wires:
  type/1 -> If/1
  If/1 -> Revolute Action/Action
  If/2 -> Prismatic Action/Action
  Revolute Action/1(J_v) -> Add/1
  Prismatic Action/1(J_v) -> Add/2
  Add/1 -> J_v/1
  R/1 -> Prismatic Action/1(R), Revolute Action/1(R)
  p/1 -> Revolute Action/2(p)
  pn/1 -> Revolute Action/3(pn)

== system Dynamics/Subsystem2/Jacobian/J(q) gen./J_v_4(q)/J_v_1 ==
  R : Inport
  p : Inport  Port=2
  pn : Inport  Port=3
  type : Inport  Port=4
  Add : Sum
  If : If  IfExpression=u1 == 1
  Prismatic Action : Subsystem  TreatAsAtomicUnit=on
  Revolute Action : Subsystem  TreatAsAtomicUnit=on
  J_v : Outport
  wires:
  type/1 -> If/1
  If/1 -> Revolute Action/Action
  If/2 -> Prismatic Action/Action
  Revolute Action/1(J_v) -> Add/1
  Prismatic Action/1(J_v) -> Add/2
  Add/1 -> J_v/1
  R/1 -> Prismatic Action/1(R), Revolute Action/1(R)
  p/1 -> Revolute Action/2(p)
  pn/1 -> Revolute Action/3(pn)

== system Dynamics/Subsystem2/Jacobian/J(q) gen./J_v_4(q)/J_v_2 ==
  R : Inport
  p : Inport  Port=2
  pn : Inport  Port=3
  type : Inport  Port=4
  Add : Sum
  If : If  IfExpression=u1 == 1
  Prismatic Action : Subsystem  TreatAsAtomicUnit=on
  Revolute Action : Subsystem  TreatAsAtomicUnit=on
  J_v : Outport
  wires:
  type/1 -> If/1
  If/1 -> Revolute Action/Action
  If/2 -> Prismatic Action/Action
  Revolute Action/1(J_v) -> Add/1
  Prismatic Action/1(J_v) -> Add/2
  Add/1 -> J_v/1
  R/1 -> Prismatic Action/1(R), Revolute Action/1(R)
  p/1 -> Revolute Action/2(p)
  pn/1 -> Revolute Action/3(pn)

== system Dynamics/Subsystem2/Jacobian/J(q) gen./J_v_4(q)/J_v_3 ==
  R : Inport
  p : Inport  Port=2
  pn : Inport  Port=3
  type : Inport  Port=4
  Add : Sum
  If : If  IfExpression=u1 == 1
  Prismatic Action : Subsystem  TreatAsAtomicUnit=on
  Revolute Action : Subsystem  TreatAsAtomicUnit=on
  J_v : Outport
  wires:
  type/1 -> If/1
  If/1 -> Revolute Action/Action
  If/2 -> Prismatic Action/Action
  Revolute Action/1(J_v) -> Add/1
  Prismatic Action/1(J_v) -> Add/2
  Add/1 -> J_v/1
  R/1 -> Prismatic Action/1(R), Revolute Action/1(R)
  p/1 -> Revolute Action/2(p)
  pn/1 -> Revolute Action/3(pn)

== system Dynamics/Subsystem2/Jacobian/J(q) gen./J_v_5(q)/J_v_1 ==
  R : Inport
  p : Inport  Port=2
  pn : Inport  Port=3
  type : Inport  Port=4
  Add : Sum
  If : If  IfExpression=u1 == 1
  Prismatic Action : Subsystem  TreatAsAtomicUnit=on
  Revolute Action : Subsystem  TreatAsAtomicUnit=on
  J_v : Outport
  wires:
  type/1 -> If/1
  If/1 -> Revolute Action/Action
  If/2 -> Prismatic Action/Action
  Revolute Action/1(J_v) -> Add/1
  Prismatic Action/1(J_v) -> Add/2
  Add/1 -> J_v/1
  R/1 -> Prismatic Action/1(R), Revolute Action/1(R)
  p/1 -> Revolute Action/2(p)
  pn/1 -> Revolute Action/3(pn)

== system Dynamics/Subsystem2/Jacobian/J(q) gen./J_v_5(q)/J_v_2 ==
  R : Inport
  p : Inport  Port=2
  pn : Inport  Port=3
  type : Inport  Port=4
  Add : Sum
  If : If  IfExpression=u1 == 1
  Prismatic Action : Subsystem  TreatAsAtomicUnit=on
  Revolute Action : Subsystem  TreatAsAtomicUnit=on
  J_v : Outport
  wires:
  type/1 -> If/1
  If/1 -> Revolute Action/Action
  If/2 -> Prismatic Action/Action
  Revolute Action/1(J_v) -> Add/1
  Prismatic Action/1(J_v) -> Add/2
  Add/1 -> J_v/1
  R/1 -> Prismatic Action/1(R), Revolute Action/1(R)
  p/1 -> Revolute Action/2(p)
  pn/1 -> Revolute Action/3(pn)

== system Dynamics/Subsystem2/Jacobian/J(q) gen./J_v_5(q)/J_v_3 ==
  R : Inport
  p : Inport  Port=2
  pn : Inport  Port=3
  type : Inport  Port=4
  Add : Sum
  If : If  IfExpression=u1 == 1
  Prismatic Action : Subsystem  TreatAsAtomicUnit=on
  Revolute Action : Subsystem  TreatAsAtomicUnit=on
  J_v : Outport
  wires:
  type/1 -> If/1
  If/1 -> Revolute Action/Action
  If/2 -> Prismatic Action/Action
  Revolute Action/1(J_v) -> Add/1
  Prismatic Action/1(J_v) -> Add/2
  Add/1 -> J_v/1
  R/1 -> Prismatic Action/1(R), Revolute Action/1(R)
  p/1 -> Revolute Action/2(p)
  pn/1 -> Revolute Action/3(pn)

== system Dynamics/Subsystem2/Jacobian/J(q) gen./J_v_5(q)/J_v_4 ==
  R : Inport
  p : Inport  Port=2
  pn : Inport  Port=3
  type : Inport  Port=4
  Add : Sum
  If : If  IfExpression=u1 == 1
  Prismatic Action : Subsystem  TreatAsAtomicUnit=on
  Revolute Action : Subsystem  TreatAsAtomicUnit=on
  J_v : Outport
  wires:
  type/1 -> If/1
  If/1 -> Revolute Action/Action
  If/2 -> Prismatic Action/Action
  Revolute Action/1(J_v) -> Add/1
  Prismatic Action/1(J_v) -> Add/2
  Add/1 -> J_v/1
  R/1 -> Prismatic Action/1(R), Revolute Action/1(R)
  p/1 -> Revolute Action/2(p)
  pn/1 -> Revolute Action/3(pn)

== system Dynamics/Subsystem2/Jacobian/J_v/J_v_1/Prismatic Action ==
  R : Inport
  Action Port : ActionPort  ActionPortLabel=else
  Constant : Constant  Value=[0;0;1]
  Product : Product  Multiplication=Matrix(*)
  J_v : Outport
  wires:
  Product/1 -> J_v/1
  R/1 -> Product/1
  Constant/1 -> Product/2

== system Dynamics/Subsystem2/Jacobian/J_v/J_v_1/Revolute Action ==
  R : Inport
  p : Inport  Port=2
  pn : Inport  Port=3
  Action Port : ActionPort  ActionPortLabel=if(u1 == 1)
  3x3 Cross Product : Subsystem  Description=Replaced Block  mask(Replaced Block){}
      mask help: This block has been replaced with an empty subsystem because it used functionality that is unavailable in Simulink R2021a.
      mask Display: fprintf('Replaced: %s\n','CrossProduct')
  Add : Sum  Inputs=-+
  Constant : Constant  Value=[0;0;1]
  Product : Product  Multiplication=Matrix(*)
  J_v : Outport
  wires:
  3x3 Cross Product/1(Out1) -> J_v/1
  p/1 -> Add/1
  pn/1 -> Add/2
  Add/1 -> 3x3 Cross Product/2(In2)
  R/1 -> Product/1
  Constant/1 -> Product/2
  Product/1 -> 3x3 Cross Product/1(In1)

== system Dynamics/Subsystem2/Jacobian/J_v/J_v_2/Prismatic Action ==
  R : Inport
  Action Port : ActionPort  ActionPortLabel=else
  Constant : Constant  Value=[0;0;1]
  Product : Product  Multiplication=Matrix(*)
  J_v : Outport
  wires:
  Product/1 -> J_v/1
  R/1 -> Product/1
  Constant/1 -> Product/2

== system Dynamics/Subsystem2/Jacobian/J_v/J_v_2/Revolute Action ==
  R : Inport
  p : Inport  Port=2
  pn : Inport  Port=3
  Action Port : ActionPort  ActionPortLabel=if(u1 == 1)
  3x3 Cross Product : Subsystem  Description=Replaced Block  mask(Replaced Block){}
      mask help: This block has been replaced with an empty subsystem because it used functionality that is unavailable in Simulink R2021a.
      mask Display: fprintf('Replaced: %s\n','CrossProduct')
  Add : Sum  Inputs=-+
  Constant : Constant  Value=[0;0;1]
  Product : Product  Multiplication=Matrix(*)
  J_v : Outport
  wires:
  3x3 Cross Product/1(Out1) -> J_v/1
  p/1 -> Add/1
  pn/1 -> Add/2
  Add/1 -> 3x3 Cross Product/2(In2)
  R/1 -> Product/1
  Constant/1 -> Product/2
  Product/1 -> 3x3 Cross Product/1(In1)

== system Dynamics/Subsystem2/Jacobian/J_v/J_v_3/Prismatic Action ==
  R : Inport
  Action Port : ActionPort  ActionPortLabel=else
  Constant : Constant  Value=[0;0;1]
  Product : Product  Multiplication=Matrix(*)
  J_v : Outport
  wires:
  Product/1 -> J_v/1
  R/1 -> Product/1
  Constant/1 -> Product/2

== system Dynamics/Subsystem2/Jacobian/J_v/J_v_3/Revolute Action ==
  R : Inport
  p : Inport  Port=2
  pn : Inport  Port=3
  Action Port : ActionPort  ActionPortLabel=if(u1 == 1)
  3x3 Cross Product : Subsystem  Description=Replaced Block  mask(Replaced Block){}
      mask help: This block has been replaced with an empty subsystem because it used functionality that is unavailable in Simulink R2021a.
      mask Display: fprintf('Replaced: %s\n','CrossProduct')
  Add : Sum  Inputs=-+
  Constant : Constant  Value=[0;0;1]
  Product : Product  Multiplication=Matrix(*)
  J_v : Outport
  wires:
  3x3 Cross Product/1(Out1) -> J_v/1
  p/1 -> Add/1
  pn/1 -> Add/2
  Add/1 -> 3x3 Cross Product/2(In2)
  R/1 -> Product/1
  Constant/1 -> Product/2
  Product/1 -> 3x3 Cross Product/1(In1)

== system Dynamics/Subsystem2/Jacobian/J_v/J_v_4/Prismatic Action ==
  R : Inport
  Action Port : ActionPort  ActionPortLabel=else
  Constant : Constant  Value=[0;0;1]
  Product : Product  Multiplication=Matrix(*)
  J_v : Outport
  wires:
  Product/1 -> J_v/1
  R/1 -> Product/1
  Constant/1 -> Product/2

== system Dynamics/Subsystem2/Jacobian/J_v/J_v_4/Revolute Action ==
  R : Inport
  p : Inport  Port=2
  pn : Inport  Port=3
  Action Port : ActionPort  ActionPortLabel=if(u1 == 1)
  3x3 Cross Product : Subsystem  Description=Replaced Block  mask(Replaced Block){}
      mask help: This block has been replaced with an empty subsystem because it used functionality that is unavailable in Simulink R2021a.
      mask Display: fprintf('Replaced: %s\n','CrossProduct')
  Add : Sum  Inputs=-+
  Constant : Constant  Value=[0;0;1]
  Product : Product  Multiplication=Matrix(*)
  J_v : Outport
  wires:
  3x3 Cross Product/1(Out1) -> J_v/1
  p/1 -> Add/1
  pn/1 -> Add/2
  Add/1 -> 3x3 Cross Product/2(In2)
  R/1 -> Product/1
  Constant/1 -> Product/2
  Product/1 -> 3x3 Cross Product/1(In1)

== system Dynamics/Subsystem2/Jacobian/J_v/J_v_5/Prismatic Action ==
  R : Inport
  Action Port : ActionPort  ActionPortLabel=else
  Constant : Constant  Value=[0;0;1]
  Product : Product  Multiplication=Matrix(*)
  J_v : Outport
  wires:
  Product/1 -> J_v/1
  R/1 -> Product/1
  Constant/1 -> Product/2

== system Dynamics/Subsystem2/Jacobian/J_v/J_v_5/Revolute Action ==
  R : Inport
  p : Inport  Port=2
  pn : Inport  Port=3
  Action Port : ActionPort  ActionPortLabel=if(u1 == 1)
  3x3 Cross Product : Subsystem  Description=Replaced Block  mask(Replaced Block){}
      mask help: This block has been replaced with an empty subsystem because it used functionality that is unavailable in Simulink R2021a.
      mask Display: fprintf('Replaced: %s\n','CrossProduct')
  Add : Sum  Inputs=-+
  Constant : Constant  Value=[0;0;1]
  Product : Product  Multiplication=Matrix(*)
  J_v : Outport
  wires:
  3x3 Cross Product/1(Out1) -> J_v/1
  p/1 -> Add/1
  pn/1 -> Add/2
  Add/1 -> 3x3 Cross Product/2(In2)
  R/1 -> Product/1
  Constant/1 -> Product/2
  Product/1 -> 3x3 Cross Product/1(In1)

== system Dynamics/Subsystem2/Jacobian/J_v/J_v_6/Prismatic Action ==
  R : Inport
  Action Port : ActionPort  ActionPortLabel=else
  Constant : Constant  Value=[0;0;1]
  Product : Product  Multiplication=Matrix(*)
  J_v : Outport
  wires:
  Product/1 -> J_v/1
  R/1 -> Product/1
  Constant/1 -> Product/2

== system Dynamics/Subsystem2/Jacobian/J_v/J_v_6/Revolute Action ==
  R : Inport
  p : Inport  Port=2
  pn : Inport  Port=3
  Action Port : ActionPort  ActionPortLabel=if(u1 == 1)
  3x3 Cross Product : Subsystem  Description=Replaced Block  mask(Replaced Block){}
      mask help: This block has been replaced with an empty subsystem because it used functionality that is unavailable in Simulink R2021a.
      mask Display: fprintf('Replaced: %s\n','CrossProduct')
  Add : Sum  Inputs=-+
  Constant : Constant  Value=[0;0;1]
  Product : Product  Multiplication=Matrix(*)
  J_v : Outport
  wires:
  3x3 Cross Product/1(Out1) -> J_v/1
  p/1 -> Add/1
  pn/1 -> Add/2
  Add/1 -> 3x3 Cross Product/2(In2)
  R/1 -> Product/1
  Constant/1 -> Product/2
  Product/1 -> 3x3 Cross Product/1(In1)

== system Dynamics/DYNAMIC/Jacobian/J(q) gen./J_v_2(q)/J_v_1/Prismatic Action ==
  R : Inport
  Action Port : ActionPort  ActionPortLabel=else
  Constant : Constant  Value=[0;0;1]
  Product : Product  Multiplication=Matrix(*)
  J_v : Outport
  wires:
  Product/1 -> J_v/1
  R/1 -> Product/1
  Constant/1 -> Product/2

== system Dynamics/DYNAMIC/Jacobian/J(q) gen./J_v_2(q)/J_v_1/Revolute Action ==
  R : Inport
  p : Inport  Port=2
  pn : Inport  Port=3
  Action Port : ActionPort  ActionPortLabel=if(u1 == 1)
  3x3 Cross Product : sharedutil/3x3 Cross Product  aMode=aMode
  Add : Sum  Inputs=-+
  Constant : Constant  Value=[0;0;1]
  Product : Product  Multiplication=Matrix(*)
  J_v : Outport
  wires:
  3x3 Cross Product/1 -> J_v/1
  p/1 -> Add/1
  pn/1 -> Add/2
  Add/1 -> 3x3 Cross Product/2
  R/1 -> Product/1
  Constant/1 -> Product/2
  Product/1 -> 3x3 Cross Product/1

== system Dynamics/DYNAMIC/Jacobian/J(q) gen./J_v_3(q)/J_v_1/Prismatic Action ==
  R : Inport
  Action Port : ActionPort  ActionPortLabel=else
  Constant : Constant  Value=[0;0;1]
  Product : Product  Multiplication=Matrix(*)
  J_v : Outport
  wires:
  Product/1 -> J_v/1
  R/1 -> Product/1
  Constant/1 -> Product/2

== system Dynamics/DYNAMIC/Jacobian/J(q) gen./J_v_3(q)/J_v_1/Revolute Action ==
  R : Inport
  p : Inport  Port=2
  pn : Inport  Port=3
  Action Port : ActionPort  ActionPortLabel=if(u1 == 1)
  3x3 Cross Product : sharedutil/3x3 Cross Product  aMode=aMode
  Add : Sum  Inputs=-+
  Constant : Constant  Value=[0;0;1]
  Product : Product  Multiplication=Matrix(*)
  J_v : Outport
  wires:
  3x3 Cross Product/1 -> J_v/1
  p/1 -> Add/1
  pn/1 -> Add/2
  Add/1 -> 3x3 Cross Product/2
  R/1 -> Product/1
  Constant/1 -> Product/2
  Product/1 -> 3x3 Cross Product/1

== system Dynamics/DYNAMIC/Jacobian/J(q) gen./J_v_3(q)/J_v_2/Prismatic Action ==
  R : Inport
  Action Port : ActionPort  ActionPortLabel=else
  Constant : Constant  Value=[0;0;1]
  Product : Product  Multiplication=Matrix(*)
  J_v : Outport
  wires:
  Product/1 -> J_v/1
  R/1 -> Product/1
  Constant/1 -> Product/2

== system Dynamics/DYNAMIC/Jacobian/J(q) gen./J_v_3(q)/J_v_2/Revolute Action ==
  R : Inport
  p : Inport  Port=2
  pn : Inport  Port=3
  Action Port : ActionPort  ActionPortLabel=if(u1 == 1)
  3x3 Cross Product : sharedutil/3x3 Cross Product  aMode=aMode
  Add : Sum  Inputs=-+
  Constant : Constant  Value=[0;0;1]
  Product : Product  Multiplication=Matrix(*)
  J_v : Outport
  wires:
  3x3 Cross Product/1 -> J_v/1
  p/1 -> Add/1
  pn/1 -> Add/2
  Add/1 -> 3x3 Cross Product/2
  R/1 -> Product/1
  Constant/1 -> Product/2
  Product/1 -> 3x3 Cross Product/1

== system Dynamics/DYNAMIC/Jacobian/J(q) gen./J_v_4(q)/J_v_1/Prismatic Action ==
  R : Inport
  Action Port : ActionPort  ActionPortLabel=else
  Constant : Constant  Value=[0;0;1]
  Product : Product  Multiplication=Matrix(*)
  J_v : Outport
  wires:
  Product/1 -> J_v/1
  R/1 -> Product/1
  Constant/1 -> Product/2

== system Dynamics/DYNAMIC/Jacobian/J(q) gen./J_v_4(q)/J_v_1/Revolute Action ==
  R : Inport
  p : Inport  Port=2
  pn : Inport  Port=3
  Action Port : ActionPort  ActionPortLabel=if(u1 == 1)
  3x3 Cross Product : sharedutil/3x3 Cross Product  aMode=aMode
  Add : Sum  Inputs=-+
  Constant : Constant  Value=[0;0;1]
  Product : Product  Multiplication=Matrix(*)
  J_v : Outport
  wires:
  3x3 Cross Product/1 -> J_v/1
  p/1 -> Add/1
  pn/1 -> Add/2
  Add/1 -> 3x3 Cross Product/2
  R/1 -> Product/1
  Constant/1 -> Product/2
  Product/1 -> 3x3 Cross Product/1

== system Dynamics/DYNAMIC/Jacobian/J(q) gen./J_v_4(q)/J_v_2/Prismatic Action ==
  R : Inport
  Action Port : ActionPort  ActionPortLabel=else
  Constant : Constant  Value=[0;0;1]
  Product : Product  Multiplication=Matrix(*)
  J_v : Outport
  wires:
  Product/1 -> J_v/1
  R/1 -> Product/1
  Constant/1 -> Product/2

== system Dynamics/DYNAMIC/Jacobian/J(q) gen./J_v_4(q)/J_v_2/Revolute Action ==
  R : Inport
  p : Inport  Port=2
  pn : Inport  Port=3
  Action Port : ActionPort  ActionPortLabel=if(u1 == 1)
  3x3 Cross Product : sharedutil/3x3 Cross Product  aMode=aMode
  Add : Sum  Inputs=-+
  Constant : Constant  Value=[0;0;1]
  Product : Product  Multiplication=Matrix(*)
  J_v : Outport
  wires:
  3x3 Cross Product/1 -> J_v/1
  p/1 -> Add/1
  pn/1 -> Add/2
  Add/1 -> 3x3 Cross Product/2
  R/1 -> Product/1
  Constant/1 -> Product/2
  Product/1 -> 3x3 Cross Product/1

== system Dynamics/DYNAMIC/Jacobian/J(q) gen./J_v_4(q)/J_v_3/Prismatic Action ==
  R : Inport
  Action Port : ActionPort  ActionPortLabel=else
  Constant : Constant  Value=[0;0;1]
  Product : Product  Multiplication=Matrix(*)
  J_v : Outport
  wires:
  Product/1 -> J_v/1
  R/1 -> Product/1
  Constant/1 -> Product/2

== system Dynamics/DYNAMIC/Jacobian/J(q) gen./J_v_4(q)/J_v_3/Revolute Action ==
  R : Inport
  p : Inport  Port=2
  pn : Inport  Port=3
  Action Port : ActionPort  ActionPortLabel=if(u1 == 1)
  3x3 Cross Product : sharedutil/3x3 Cross Product  aMode=aMode
  Add : Sum  Inputs=-+
  Constant : Constant  Value=[0;0;1]
  Product : Product  Multiplication=Matrix(*)
  J_v : Outport
  wires:
  3x3 Cross Product/1 -> J_v/1
  p/1 -> Add/1
  pn/1 -> Add/2
  Add/1 -> 3x3 Cross Product/2
  R/1 -> Product/1
  Constant/1 -> Product/2
  Product/1 -> 3x3 Cross Product/1

== system Dynamics/DYNAMIC/Jacobian/J(q) gen./J_v_5(q)/J_v_1/Prismatic Action ==
  R : Inport
  Action Port : ActionPort  ActionPortLabel=else
  Constant : Constant  Value=[0;0;1]
  Product : Product  Multiplication=Matrix(*)
  J_v : Outport
  wires:
  Product/1 -> J_v/1
  R/1 -> Product/1
  Constant/1 -> Product/2

== system Dynamics/DYNAMIC/Jacobian/J(q) gen./J_v_5(q)/J_v_1/Revolute Action ==
  R : Inport
  p : Inport  Port=2
  pn : Inport  Port=3
  Action Port : ActionPort  ActionPortLabel=if(u1 == 1)
  3x3 Cross Product : sharedutil/3x3 Cross Product  aMode=aMode
  Add : Sum  Inputs=-+
  Constant : Constant  Value=[0;0;1]
  Product : Product  Multiplication=Matrix(*)
  J_v : Outport
  wires:
  3x3 Cross Product/1 -> J_v/1
  p/1 -> Add/1
  pn/1 -> Add/2
  Add/1 -> 3x3 Cross Product/2
  R/1 -> Product/1
  Constant/1 -> Product/2
  Product/1 -> 3x3 Cross Product/1

== system Dynamics/DYNAMIC/Jacobian/J(q) gen./J_v_5(q)/J_v_2/Prismatic Action ==
  R : Inport
  Action Port : ActionPort  ActionPortLabel=else
  Constant : Constant  Value=[0;0;1]
  Product : Product  Multiplication=Matrix(*)
  J_v : Outport
  wires:
  Product/1 -> J_v/1
  R/1 -> Product/1
  Constant/1 -> Product/2
